simulink model "intento_50metrosporsegundo"  (R2024b)
settings: Solver=VariableStepAuto  StartTime=0.0  StopTime=600  RelTol=1e-3
libraries: slpidlib x1
settings Model: Creator=aulasingenieria  LastModifiedBy=Lenovo 618918
settings DebuggingCC: AlgebraicLoopMsg=none
settings RTWCC: GPUComputeCapability=3.5

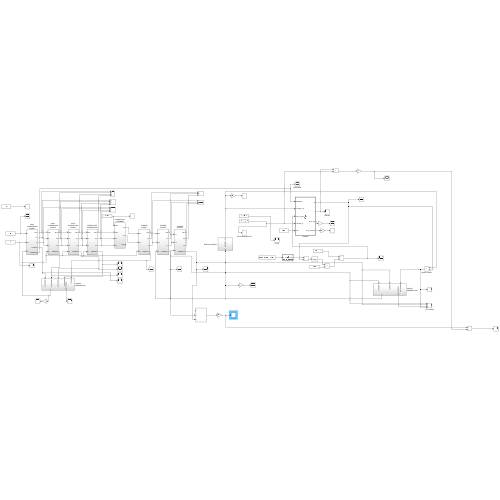
[thumbnail: Simulink's stored preview of the top-level diagram]
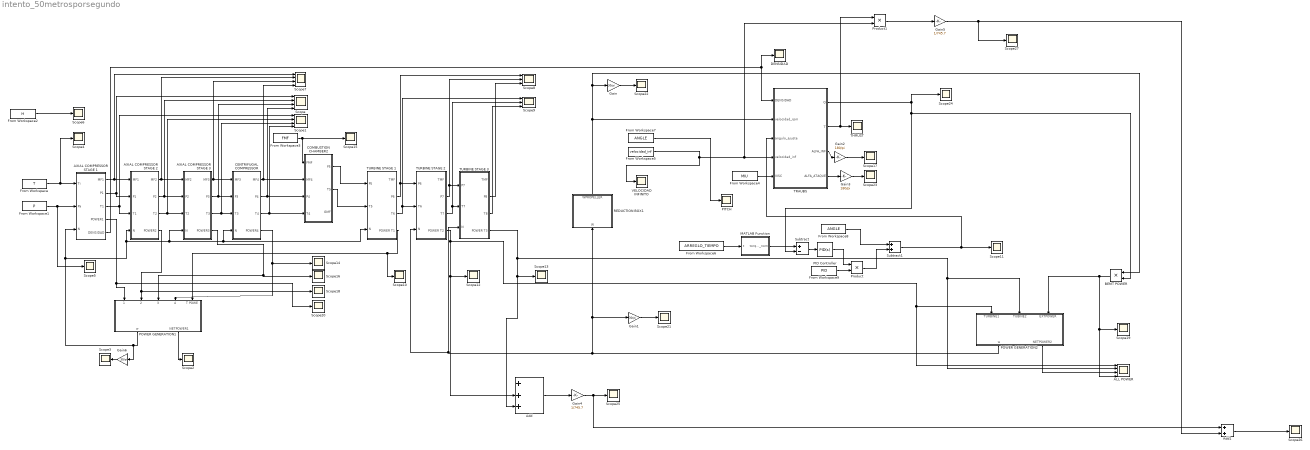
== system intento_50metrosporsegundo ==
  ALL POWER : Scope  NumInputPorts=4
  AXIAL COMPRESSOR STAGE 1 : Subsystem
  AXIAL COMPRESSOR STAGE 2 : Subsystem
  AXIAL COMPRESSOR STAGE 3 : Subsystem
  Add : Sum  Inputs=+++
  Add1 : Sum
  BEMT POWER : Product
  CENTRIFUGAL COMPRESSOR : Subsystem
  COMBUSTION CHAMBER2 : Subsystem
  DENSIDAD : Scope
  From Workspace : FromWorkspace  VariableName=T
  From Workspace1 : FromWorkspace  VariableName=P
  From Workspace2 : FromWorkspace  VariableName=H
  From Workspace3 : FromWorkspace  VariableName=FMF
  From Workspace4 : FromWorkspace  VariableName=MIU
  From Workspace5 : FromWorkspace  VariableName=velocidad_inf
  From Workspace6 : FromWorkspace  VariableName=ARREGLO_TIEMPO
  From Workspace7 : FromWorkspace  VariableName=ANGLE
  From Workspace8 : FromWorkspace  VariableName=ANGLE
  From Workspace9 : FromWorkspace  VariableName=PID
  Gain : Gain  Gain=30/pi
  Gain1 : Gain  Gain=30/pi
  Gain2 : Gain  Gain=180/pi
  Gain3 : Gain  Gain=180/pi
  Gain4 : Gain  Gain=1/745.7
  Gain5 : Gain  Gain=1/745.7
  Gain6 : Gain  Gain=30/pi
  MATLAB Function : MATLAB Function  TreatAsAtomicUnit=on
  PID Controller : slpidlib/PID Controller  Controller=PID  Form=Parallel  TimeDomain=Continuous-time  UseExternalTs=off  SampleTime=-1  IntegratorMethod=Forward Euler  FilterMethod=Forward Euler  ControllerParametersSource=internal  P=0.001  I=0.0001  UseKiTs=off  D=0.0001  UseExternalDerivativeSource=off  N=100  UseFilter=on  TunerSelectOption=Transfer Function Based (PID Tuner App)  InitialConditionSource=internal  InitialConditionForIntegrator=0  InitialConditionForFilter=0  DifferentiatorICPrevScaledInput=0  ExternalReset=none  TrackingMode=off  Kt=1  LimitOutput=off  SatLimitsSource=internal  UpperSaturationLimit=inf  LowerSaturationLimit=-inf  LinearizeAsGain=on  AntiWindupMode=none  Kb=1  LimitIntegrator=off  UpperIntegratorSaturationLimit=inf  LowerIntegratorSaturationLimit=-inf  POutMin=[]  POutMax=[]  IOutMin=[]  IOutMax=[]  DOutMin=[]  DOutMax=[]  NOutMin=[]  NOutMax=[]  SumOutMin=[]  SumOutMax=[]  SaturationOutMin=[]  SaturationOutMax=[]  PParamMin=[]  PParamMax=[]  IParamMin=[]  IParamMax=[]  DParamMin=[]  DParamMax=[]  NParamMin=[]  NParamMax=[]  KbParamMin=[]  KbParamMax=[]  KtParamMin=[]  KtParamMax=[]  KbOutMin=[]  KbOutMax=[]  KtOutMin=[]  KtOutMax=[]  IntegratorOutMin=[]  IntegratorOutMax=[]  FilterOutMin=[]  FilterOutMax=[]  SumI1OutMin=[]  SumI1OutMax=[]  SumI2OutMin=[]  SumI2OutMax=[]  SumI3OutMin=[]  SumI3OutMax=[]  SumI4OutMin=[]  SumI4OutMax=[]  SumDOutMin=[]  SumDOutMax=[]  DifferentiatorOutMin=[]  DifferentiatorOutMax=[]  FilterDiffOutCoefMin=[]  FilterDiffOutCoefMax=[]  ReciprocalOutMin=[]  ReciprocalOutMax=[]  SumDenOutMin=[]  SumDenOutMax=[]  SumNumOutMin=[]  SumNumOutMax=[]  DivideOutMin=[]  DivideOutMax=[]  UdiffTsProdOutMin=[]  UdiffTsProdOutMax=[]  NTsProdOutMin=[]  NTsProdOutMax=[]  UintegralTsProdOutMin=[]  UintegralTsProdOutMax=[]  UngainTsProdOutMin=[]  UngainTsProdOutMax=[]  ClampingZeroOutDataTypeStr=Inherit: Inherit via back propagation  ClampingZeroOutMin=[]  ClampingZeroOutMax=[]  FilterDenConstantOutDataTypeStr=Inherit: Inherit via back propagation  FilterDenConstantOutMin=[]  FilterDenConstantOutMax=[]  PCopyOutDataTypeStr=Inherit: Inherit via back propagation  PCopyOutMin=[]  PCopyOutMax=[]  NCopyOutDataTypeStr=Inherit: Inherit via back propagation  NCopyOutMin=[]  NCopyOutMax=[]  IntegratorContinuousStateAttributes=''  IntegratorStateMustResolveToSignalObject=off  IntegratorRTWStateStorageClass=Auto  FilterContinuousStateAttributes=''  FilterStateMustResolveToSignalObject=off  FilterRTWStateStorageClass=Auto  ParallelPVariant=InternalParameters  IdealPVariant=Disabled  IVariant=InternalParameters  DVariant=InternalParameters  IntegratorVariant=Continuous  SatVariant=Disabled  AWVariant=Passthrough  PCopyVariant=Disabled  TRVariant=Disabled  FdbkBlocksVariant=Forward  IdealPFdbkVariant=Disabled  SatFdbkVariant=Disabled  DerivativeFilterVariant=ContFilter  NVariant=InternalParameters  NCopyVariant=Disabled  FilterICVariant=InternalICsFilter  IntegratorICVariant=InternalICs  ExternalResetVariant=Disabled  TRSumVariant=Passthrough  SumFdbkVariant=Disabled  SumVariant=Sum_PID  TsampFilterVariant=InternalTs  TsampNgainVariant=Passthrough  TsampIntegralVariant=Disabled_SignalSpec  ExternalSaturationOutDataTypeStr=Inherit: Same as second input  DerivativeSourceVariant=ErrorSignal  PreIntVariant=InternalPreInt
  PITCH : Scope
  POWER GENERATION1 : Subsystem
  POWER GENERATION2 : Subsystem
  Product : Product
  Product1 : Product
  REDUCTION BOX1 : Subsystem
  Scope : Scope  NumInputPorts=4
  Scope1 : Scope  NumInputPorts=4
  Scope{2..6,10..27} (23 alike) : Scope
  Scope7 : Scope  NumInputPorts=4
  Scope8 : Scope  NumInputPorts=3
  Scope9 : Scope  NumInputPorts=3
  Subtract : Sum  Inputs=+-
  Subtract1 : Sum
  THRUST : Scope
  TRAUBS : MATLAB Function  TreatAsAtomicUnit=on
  TURBINE STAGE 1 : Subsystem
  TURBINE STAGE 2 : Subsystem
  TURBINE STAGE 3 : Subsystem
  VELOCIDAD INFINITO : Scope
  wires:
  TURBINE STAGE 1/2(P6) -> Scope8/1, TURBINE STAGE 2/1(P6)
  TURBINE STAGE 2/3(T7) -> TURBINE STAGE 3/2(T7), Scope9/2
  AXIAL COMPRESSOR STAGE 3/3(T3) -> CENTRIFUGAL COMPRESSOR/3(T3), Scope1/3
  CENTRIFUGAL COMPRESSOR/4(POWER4) -> POWER GENERATION1/4(CC POWER), Scope14/1
  CENTRIFUGAL COMPRESSOR/2(P4) -> COMBUSTION CHAMBER2/3(P4), Scope/4
  TURBINE STAGE 2/2(P7) -> Scope8/2, TURBINE STAGE 3/1(P7)
  TURBINE STAGE 3/2(P8) -> Scope8/3
  AXIAL COMPRESSOR STAGE 3/1(MF3) -> CENTRIFUGAL COMPRESSOR/1(MF3), Scope7/3
  TURBINE STAGE 3/3(T8) -> Scope9/3
  CENTRIFUGAL COMPRESSOR/3(T4) -> COMBUSTION CHAMBER2/4(T4), Scope1/4
  AXIAL COMPRESSOR STAGE 2/2(P2) -> AXIAL COMPRESSOR STAGE 3/2(P2), Scope/2
  TURBINE STAGE 1/3(T6) -> TURBINE STAGE 2/2(T6), Scope9/1
  POWER GENERATION1/1(w) -> Gain6/1, AXIAL COMPRESSOR STAGE 1/3(N), AXIAL COMPRESSOR STAGE 3/4(N), CENTRIFUGAL COMPRESSOR/4(N), TURBINE STAGE 1/3(N), AXIAL COMPRESSOR STAGE 2/4(N)
  AXIAL COMPRESSOR STAGE 3/2(P3) -> CENTRIFUGAL COMPRESSOR/2(P3), Scope/3
  From Workspace1/1 -> Scope5/1, AXIAL COMPRESSOR STAGE 1/2(Pa)
  CENTRIFUGAL COMPRESSOR/1(MF4) -> Scope7/4, COMBUSTION CHAMBER2/2(MF4)
  COMBUSTION CHAMBER2/1(P5) -> TURBINE STAGE 1/1(P5)
  POWER GENERATION1/2(NETPOWER1) -> Scope2/1
  AXIAL COMPRESSOR STAGE 2/1(MF2) -> AXIAL COMPRESSOR STAGE 3/1(MF2), Scope7/2
  From Workspace3/1 -> Scope15/1, COMBUSTION CHAMBER2/1(FMF)
  AXIAL COMPRESSOR STAGE 3/4(POWER3) -> Scope16/1, POWER GENERATION1/3(AC POWER3)
  AXIAL COMPRESSOR STAGE 2/3(T2) -> AXIAL COMPRESSOR STAGE 3/3(T2), Scope1/2
  TURBINE STAGE 1/4(POWER T1) -> Scope10/1, POWER GENERATION1/5(T POWE)
  AXIAL COMPRESSOR STAGE 1/2(P1) -> AXIAL COMPRESSOR STAGE 2/2(P1), Scope/1
  AXIAL COMPRESSOR STAGE 1/1(MF1) -> AXIAL COMPRESSOR STAGE 2/1(MF1), Scope7/1
  AXIAL COMPRESSOR STAGE 2/4(POWER2) -> Scope18/1, POWER GENERATION1/2(AC POWER2)
  From Workspace/1 -> Scope4/1, AXIAL COMPRESSOR STAGE 1/1(Ti)
  AXIAL COMPRESSOR STAGE 1/4(POWER1) -> Scope20/1, POWER GENERATION1/1(AC POWER1)
  AXIAL COMPRESSOR STAGE 1/3(T1) -> AXIAL COMPRESSOR STAGE 2/3(T1), Scope1/1
  COMBUSTION CHAMBER2/2(T5) -> TURBINE STAGE 1/2(T5)
  From Workspace2/1 -> Scope6/1
  TURBINE STAGE 2/4(POWER T2) -> Scope12/1, Add/2, ALL POWER/1, POWER GENERATION2/1(TURBINE1)
  TURBINE STAGE 3/4(POWER T3) -> Add/3, Scope13/1, ALL POWER/2, POWER GENERATION2/2(TUBINE2)
  From Workspace5/1 -> Product1/2, TRAUBS/4(velocidad_inf), VELOCIDAD INFINITO/1
  POWER GENERATION2/2(NETPOWER2) -> ALL POWER/3
  Gain/1 -> Scope22/1
  REDUCTION BOX1/1(WPROPELLER) -> BEMT POWER/1, Gain/1, TRAUBS/2(velocidad_rpm)
  BEMT POWER/1 -> POWER GENERATION2/3(EXTPOWER), Scope19/1, ALL POWER/4
  AXIAL COMPRESSOR STAGE 1/5(DENSIDAD) -> DENSIDAD/1, TRAUBS/1(DENSIDAD)
  From Workspace4/1 -> TRAUBS/5(VISC)
  Subtract/1 -> PID Controller/1
  MATLAB Function/1(torque_nom) -> Subtract/1
  From Workspace6/1 -> MATLAB Function/1(t)
  From Workspace8/1 -> Subtract1/1
  POWER GENERATION2/1(w) -> Gain1/1, REDUCTION BOX1/1(W), TURBINE STAGE 3/3(N), TURBINE STAGE 2/3(N)
  From Workspace7/1 -> PITCH/1
  TRAUBS/1(Q) -> Scope24/1, BEMT POWER/2, Subtract/2
  TRAUBS/2(T) -> Product1/1, THRUST/1
  From Workspace9/1 -> Product/2
  PID Controller/1 -> Product/1
  Product/1 -> Subtract1/2
  Gain1/1 -> Scope21/1
  TRAUBS/3(ALFA_INF) -> Gain2/1
  Gain2/1 -> Scope17/1
  TRAUBS/4(ALFA_ATAQUE) -> Gain3/1
  Gain3/1 -> Scope23/1
  Subtract1/1 -> TRAUBS/3(angulo_ajuste), Scope11/1
  Gain4/1 -> Scope25/1, Add1/1
  Add/1 -> Gain4/1
  Product1/1 -> Gain5/1
  Gain5/1 -> Scope27/1, Add1/2
  Add1/1 -> Scope26/1
  Gain6/1 -> Scope3/1

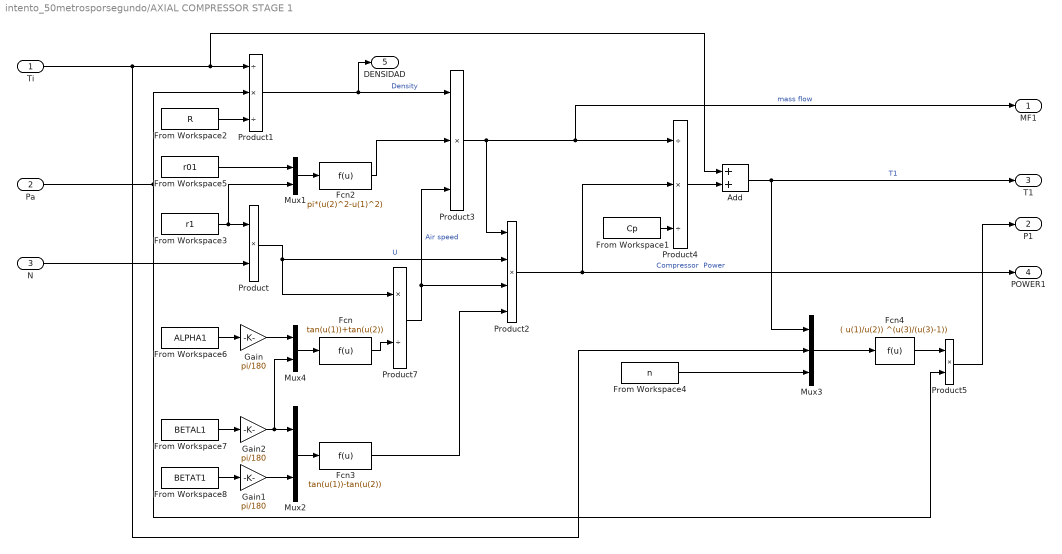
== system intento_50metrosporsegundo/AXIAL COMPRESSOR STAGE 1 ==
  Ti : Inport
  Pa : Inport  Port=2
  N : Inport  Port=3
  Add : Sum
  Fcn : Fcn  Expr=tan(u(1))+tan(u(2))
  Fcn2 : Fcn  Expr=pi*(u(2)^2-u(1)^2)
  Fcn3 : Fcn  Expr=tan(u(1))-tan(u(2))
  Fcn4 : Fcn  Expr=( u(1)/u(2)) ^(u(3)/(u(3)-1))
  From Workspace1 : FromWorkspace  VariableName=Cp
  From Workspace2 : FromWorkspace  VariableName=R
  From Workspace3 : FromWorkspace  VariableName=r1
  From Workspace4 : FromWorkspace  VariableName=n
  From Workspace5 : FromWorkspace  VariableName=r01
  From Workspace6 : FromWorkspace  VariableName=ALPHA1
  From Workspace7 : FromWorkspace  VariableName=BETAL1
  From Workspace8 : FromWorkspace  VariableName=BETAT1
  Gain : Gain  Gain=pi/180
  Gain1 : Gain  Gain=pi/180
  Gain2 : Gain  Gain=pi/180
  Mux1 : Mux  Inputs=2
  Mux2 : Mux  Inputs=2
  Mux3 : Mux  Inputs=3
  Mux4 : Mux  Inputs=2
  Product : Product
  Product1 : Product  Inputs=/*/
  Product2 : Product  Inputs=****
  Product3 : Product  Inputs=3
  Product4 : Product  Inputs=/*/
  Product5 : Product
  Product7 : Product  Inputs=*/
  MF1 : Outport
  P1 : Outport  Port=2
  T1 : Outport  Port=3
  POWER1 : Outport  Port=4
  DENSIDAD : Outport  Port=5
  wires:
  Fcn3/1 -> Product2/4
  From Workspace1/1 -> Product4/3
  Ti/1 -> Add/1, Product1/1, Mux3/2
  Mux3/1 -> Fcn4/1
  From Workspace8/1 -> Gain1/1
  Product1/1 -> DENSIDAD/1, Product3/1  "Density"
  Gain/1 -> Mux4/1
  From Workspace4/1 -> Mux3/3
  Mux1/1 -> Fcn2/1
  Mux2/1 -> Fcn3/1
  Product7/1 -> Product2/3, Product3/3  "Air speed"
  Product/1 -> Product7/1, Product2/2  "U"
  Product3/1 -> Product4/1, MF1/1, Product2/1  "mass flow"
  Fcn2/1 -> Product3/2
  Gain1/1 -> Mux2/2
  From Workspace6/1 -> Gain/1
  From Workspace5/1 -> Mux1/1
  N/1 -> Product/2
  From Workspace7/1 -> Gain2/1
  From Workspace3/1 -> Mux1/2, Product/1
  Add/1 -> T1/1, Mux3/1  "T1"
  Product4/1 -> Add/2
  From Workspace2/1 -> Product1/3
  Gain2/1 -> Mux2/1, Mux4/2
  Product2/1 -> POWER1/1, Product4/2  "Compressor  Power"
  Mux4/1 -> Fcn/1
  Product5/1 -> P1/1
  Fcn4/1 -> Product5/1
  Fcn/1 -> Product7/2
  Pa/1 -> Product1/2, Product5/2

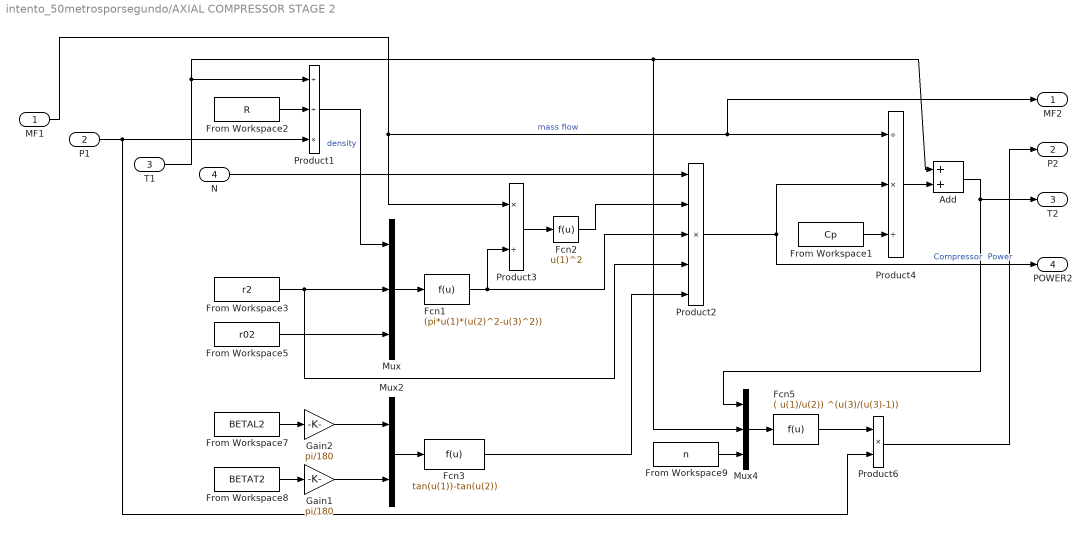
== system intento_50metrosporsegundo/AXIAL COMPRESSOR STAGE 2 ==
  MF1 : Inport
  P1 : Inport  Port=2
  T1 : Inport  Port=3
  N : Inport  Port=4
  Add : Sum
  Fcn1 : Fcn  Expr=(pi*u(1)*(u(2)^2-u(3)^2))
  Fcn2 : Fcn  Expr=u(1)^2
  Fcn3 : Fcn  Expr=tan(u(1))-tan(u(2))
  Fcn5 : Fcn  Expr=( u(1)/u(2)) ^(u(3)/(u(3)-1))
  From Workspace1 : FromWorkspace  VariableName=Cp
  From Workspace2 : FromWorkspace  VariableName=R
  From Workspace3 : FromWorkspace  VariableName=r2
  From Workspace5 : FromWorkspace  VariableName=r02
  From Workspace7 : FromWorkspace  VariableName=BETAL2
  From Workspace8 : FromWorkspace  VariableName=BETAT2
  From Workspace9 : FromWorkspace  VariableName=n
  Gain1 : Gain  Gain=pi/180
  Gain2 : Gain  Gain=pi/180
  Mux : Mux  Inputs=3
  Mux2 : Mux  Inputs=2
  Mux4 : Mux  Inputs=3
  Product1 : Product  Inputs=//*
  Product2 : Product  Inputs=*****
  Product3 : Product  Inputs=*/
  Product4 : Product  Inputs=/*/
  Product6 : Product
  MF2 : Outport
  P2 : Outport  Port=2
  T2 : Outport  Port=3
  POWER2 : Outport  Port=4
  wires:
  Add/1 -> T2/1, Mux4/1
  Product4/1 -> Add/2
  From Workspace3/1 -> Product2/4, Mux/2
  P1/1 -> Product1/3, Product6/2
  Product2/1 -> POWER2/1, Product4/2  "Compressor  Power"
  MF1/1 -> Product3/1, MF2/1, Product4/1  "mass flow"
  From Workspace5/1 -> Mux/3
  T1/1 -> Product1/1, Mux4/2, Add/1
  Fcn3/1 -> Product2/5
  From Workspace7/1 -> Gain2/1
  From Workspace1/1 -> Product4/3
  Gain2/1 -> Mux2/1
  Mux2/1 -> Fcn3/1
  Gain1/1 -> Mux2/2
  From Workspace8/1 -> Gain1/1
  From Workspace2/1 -> Product1/2
  Product1/1 -> Mux/1  "density"
  Fcn2/1 -> Product2/2
  Mux/1 -> Fcn1/1
  Fcn1/1 -> Product2/3, Product3/2
  Product3/1 -> Fcn2/1
  N/1 -> Product2/1
  Fcn5/1 -> Product6/1
  Mux4/1 -> Fcn5/1
  Product6/1 -> P2/1
  From Workspace9/1 -> Mux4/3

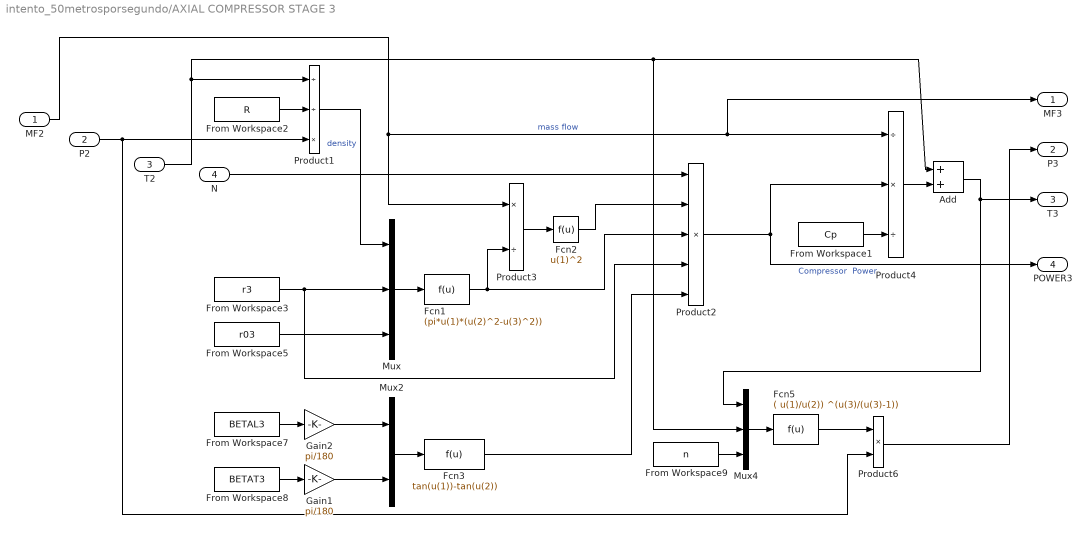
== system intento_50metrosporsegundo/AXIAL COMPRESSOR STAGE 3 ==
  MF2 : Inport
  P2 : Inport  Port=2
  T2 : Inport  Port=3
  N : Inport  Port=4
  Add : Sum
  Fcn1 : Fcn  Expr=(pi*u(1)*(u(2)^2-u(3)^2))
  Fcn2 : Fcn  Expr=u(1)^2
  Fcn3 : Fcn  Expr=tan(u(1))-tan(u(2))
  Fcn5 : Fcn  Expr=( u(1)/u(2)) ^(u(3)/(u(3)-1))
  From Workspace1 : FromWorkspace  VariableName=Cp
  From Workspace2 : FromWorkspace  VariableName=R
  From Workspace3 : FromWorkspace  VariableName=r3
  From Workspace5 : FromWorkspace  VariableName=r03
  From Workspace7 : FromWorkspace  VariableName=BETAL3
  From Workspace8 : FromWorkspace  VariableName=BETAT3
  From Workspace9 : FromWorkspace  VariableName=n
  Gain1 : Gain  Gain=pi/180
  Gain2 : Gain  Gain=pi/180
  Mux : Mux  Inputs=3
  Mux2 : Mux  Inputs=2
  Mux4 : Mux  Inputs=3
  Product1 : Product  Inputs=//*
  Product2 : Product  Inputs=*****
  Product3 : Product  Inputs=*/
  Product4 : Product  Inputs=/*/
  Product6 : Product
  MF3 : Outport
  P3 : Outport  Port=2
  T3 : Outport  Port=3
  POWER3 : Outport  Port=4
  wires:
  Add/1 -> T3/1, Mux4/1
  Product4/1 -> Add/2
  From Workspace3/1 -> Product2/4, Mux/2
  P2/1 -> Product1/3, Product6/2
  Product2/1 -> POWER3/1, Product4/2  "Compressor  Power"
  MF2/1 -> Product3/1, MF3/1, Product4/1  "mass flow"
  From Workspace5/1 -> Mux/3
  T2/1 -> Product1/1, Mux4/2, Add/1
  Fcn3/1 -> Product2/5
  From Workspace7/1 -> Gain2/1
  From Workspace1/1 -> Product4/3
  Gain2/1 -> Mux2/1
  Mux2/1 -> Fcn3/1
  Gain1/1 -> Mux2/2
  From Workspace8/1 -> Gain1/1
  From Workspace2/1 -> Product1/2
  Product1/1 -> Mux/1  "density"
  Fcn2/1 -> Product2/2
  Mux/1 -> Fcn1/1
  Fcn1/1 -> Product2/3, Product3/2
  Product3/1 -> Fcn2/1
  N/1 -> Product2/1
  Fcn5/1 -> Product6/1
  Mux4/1 -> Fcn5/1
  Product6/1 -> P3/1
  From Workspace9/1 -> Mux4/3

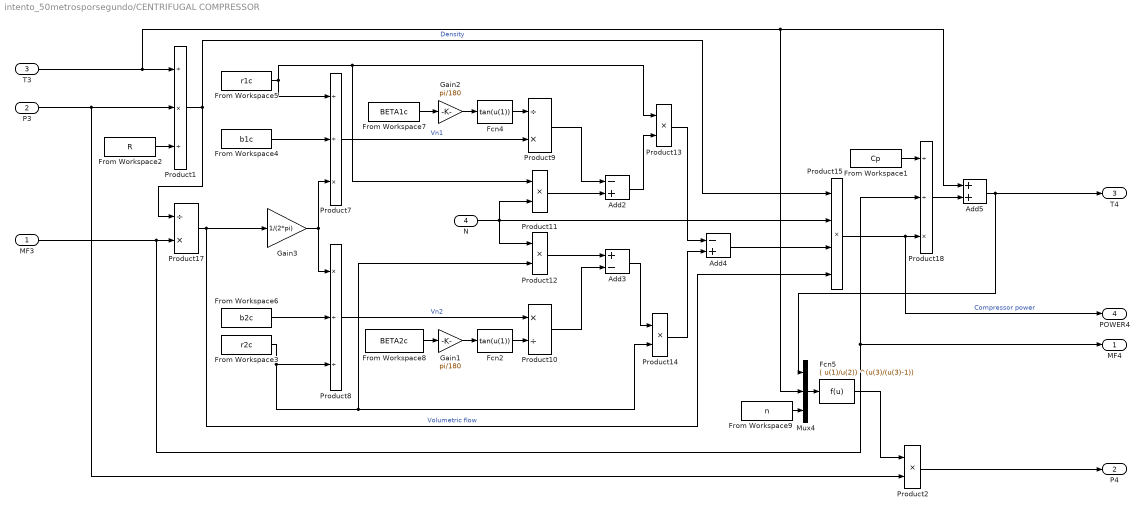
== system intento_50metrosporsegundo/CENTRIFUGAL COMPRESSOR ==
  MF3 : Inport
  P3 : Inport  Port=2
  T3 : Inport  Port=3
  N : Inport  Port=4
  Add2 : Sum  Inputs=-+
  Add3 : Sum  Inputs=+-
  Add4 : Sum  Inputs=-+
  Add5 : Sum  Inputs=2
  Fcn2 : Fcn  Expr=tan(u(1))
  Fcn4 : Fcn  Expr=tan(u(1))
  Fcn5 : Fcn  Expr=( u(1)/u(2)) ^(u(3)/(u(3)-1))
  From Workspace1 : FromWorkspace  VariableName=Cp
  From Workspace2 : FromWorkspace  VariableName=R
  From Workspace3 : FromWorkspace  VariableName=r2c
  From Workspace4 : FromWorkspace  VariableName=b1c
  From Workspace5 : FromWorkspace  VariableName=r1c
  From Workspace6 : FromWorkspace  VariableName=b2c
  From Workspace7 : FromWorkspace  VariableName=BETA1c
  From Workspace8 : FromWorkspace  VariableName=BETA2c
  From Workspace9 : FromWorkspace  VariableName=n
  Gain1 : Gain  Gain=pi/180
  Gain2 : Gain  Gain=pi/180
  Gain3 : Gain  Gain=1/(2*pi)
  Mux4 : Mux  Inputs=3
  Product1 : Product  Inputs=/*/
  Product10 : Product  Inputs=*/
  Product{2,11..14} (5 alike) : Product
  Product15 : Product  Inputs=4
  Product17 : Product  Inputs=/*
  Product18 : Product  Inputs=//*
  Product7 : Product  Inputs=//*
  Product8 : Product  Inputs=*//
  Product9 : Product  Inputs=/*
  MF4 : Outport
  P4 : Outport  Port=2
  T4 : Outport  Port=3
  POWER4 : Outport  Port=4
  wires:
  From Workspace2/1 -> Product1/3
  P3/1 -> Product1/2, Product2/2
  T3/1 -> Product1/1, Mux4/2, Add5/1
  From Workspace8/1 -> Gain1/1
  From Workspace7/1 -> Gain2/1
  From Workspace4/1 -> Product7/2
  From Workspace5/1 -> Product13/1, Product11/1, Product7/1
  Product1/1 -> Product15/1, Product17/1  "Density"
  From Workspace6/1 -> Product8/2
  Gain1/1 -> Fcn2/1
  Gain2/1 -> Fcn4/1
  Fcn4/1 -> Product9/1
  Product7/1 -> Product9/2  "Vn1"
  Product8/1 -> Product10/1  "Vn2"
  Fcn2/1 -> Product10/2
  Product10/1 -> Add3/2
  Product9/1 -> Add2/1
  N/1 -> Product12/1, Product15/2, Product11/2
  Product11/1 -> Add2/2
  Product12/1 -> Add3/1
  Add2/1 -> Product13/2
  Add3/1 -> Product14/1
  From Workspace3/1 -> Product12/2, Product14/2, Product8/3
  Product13/1 -> Add4/1
  Product14/1 -> Add4/2
  Add4/1 -> Product15/3
  Product17/1 -> Product15/4, Gain3/1  "Volumetric flow"
  MF3/1 -> Product18/2, MF4/1, Product17/2
  Gain3/1 -> Product7/3, Product8/1
  Product2/1 -> P4/1
  Product15/1 -> POWER4/1, Product18/3  "Compressor power"
  Product18/1 -> Add5/2
  From Workspace1/1 -> Product18/1
  Add5/1 -> Mux4/1, T4/1
  Mux4/1 -> Fcn5/1
  From Workspace9/1 -> Mux4/3
  Fcn5/1 -> Product2/1

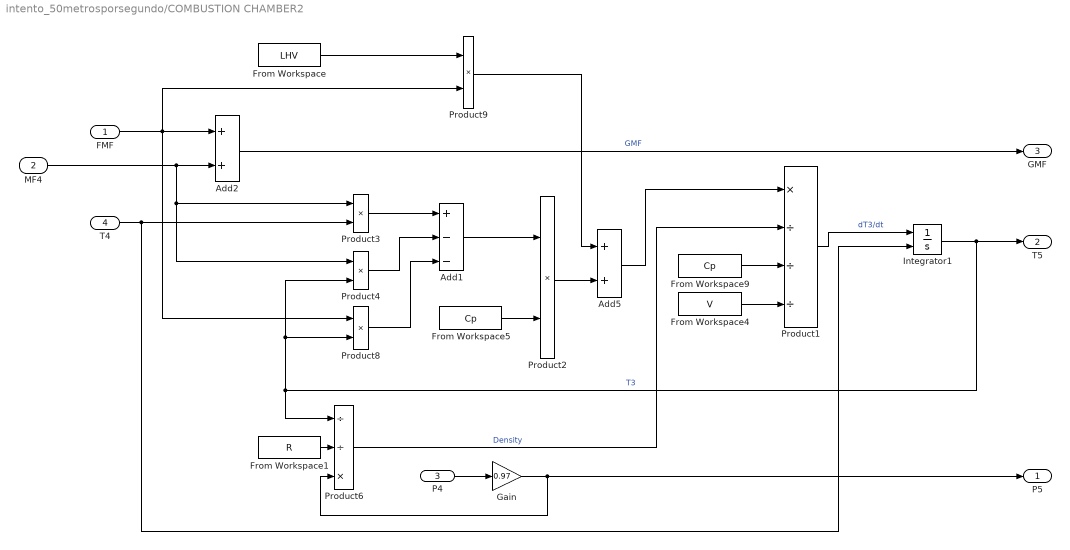
== system intento_50metrosporsegundo/COMBUSTION CHAMBER2 ==
  FMF : Inport
  MF4 : Inport  Port=2
  P4 : Inport  Port=3
  T4 : Inport  Port=4
  Add1 : Sum  Inputs=+--
  Add2 : Sum  Inputs=2
  Add5 : Sum  Inputs=2
  From Workspace : FromWorkspace  VariableName=LHV
  From Workspace1 : FromWorkspace  VariableName=R
  From Workspace4 : FromWorkspace  VariableName=V
  From Workspace5 : FromWorkspace  VariableName=Cp
  From Workspace9 : FromWorkspace  VariableName=Cp
  Gain : Gain  Gain=0.97
  Integrator1 : Integrator  InitialConditionSource=external
  Product1 : Product  Inputs=*///
  Product{2..4,8..9} (5 alike) : Product
  Product6 : Product  Inputs=//*
  P5 : Outport
  T5 : Outport  Port=2
  GMF : Outport  Port=3
  wires:
  T4/1 -> Integrator1/2, Product3/2
  Product6/1 -> Product1/2  "Density"
  MF4/1 -> Add2/2, Product3/1, Product4/1
  FMF/1 -> Add2/1, Product9/2, Product8/1
  From Workspace/1 -> Product9/1
  From Workspace4/1 -> Product1/4
  From Workspace9/1 -> Product1/3
  From Workspace5/1 -> Product2/2
  Add1/1 -> Product2/1
  Product3/1 -> Add1/1
  Product4/1 -> Add1/2
  Integrator1/1 -> Product6/1, Product8/2, Product4/2, T5/1  "T3"
  Product8/1 -> Add1/3
  Product9/1 -> Add5/1
  Product2/1 -> Add5/2
  Add5/1 -> Product1/1
  Product1/1 -> Integrator1/1  "dT3/dt"
  From Workspace1/1 -> Product6/2
  Gain/1 -> Product6/3, P5/1
  P4/1 -> Gain/1
  Add2/1 -> GMF/1  "GMF"

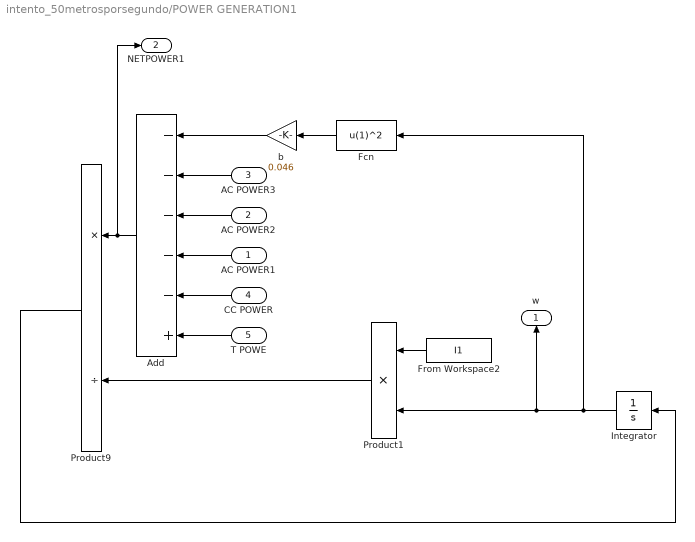
== system intento_50metrosporsegundo/POWER GENERATION1 ==
  AC POWER1 : Inport
  AC POWER2 : Inport  Port=2
  AC POWER3 : Inport  Port=3
  CC POWER : Inport  Port=4
  T POWE : Inport  Port=5
  Add : Sum  Inputs=-----+
  Fcn : Fcn  Expr=u(1)^2
  From Workspace2 : FromWorkspace  VariableName=I1
  Integrator : Integrator  InitialCondition=1256
  Product1 : Product
  Product9 : Product  Inputs=*/
  b : Gain  Gain=0.046
  w : Outport
  NETPOWER1 : Outport  Port=2
  wires:
  Product1/1 -> Product9/2
  Add/1 -> NETPOWER1/1, Product9/1
  Product9/1 -> Integrator/1
  T POWE/1 -> Add/6
  AC POWER1/1 -> Add/4
  AC POWER2/1 -> Add/3
  AC POWER3/1 -> Add/2
  CC POWER/1 -> Add/5
  From Workspace2/1 -> Product1/1
  Integrator/1 -> Fcn/1, Product1/2, w/1
  Fcn/1 -> b/1
  b/1 -> Add/1

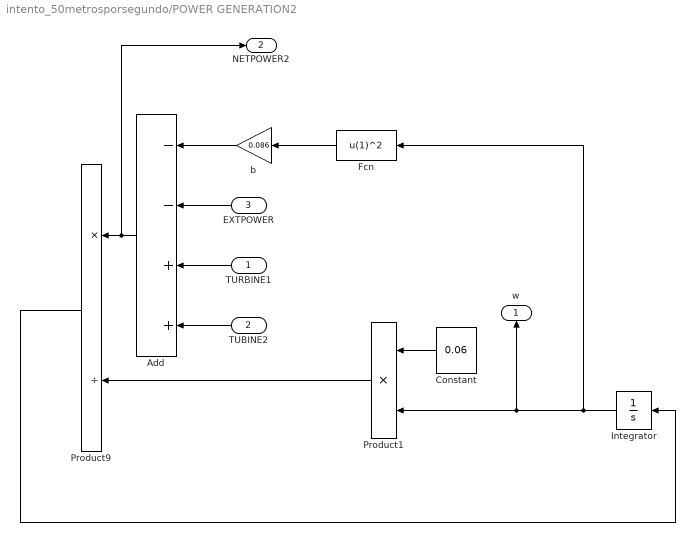
== system intento_50metrosporsegundo/POWER GENERATION2 ==
  TURBINE1 : Inport
  TUBINE2 : Inport  Port=2
  EXTPOWER : Inport  Port=3
  Add : Sum  Inputs=--++
  Constant : Constant  Value=0.06
  Fcn : Fcn  Expr=u(1)^2
  Integrator : Integrator  InitialCondition=90
  Product1 : Product
  Product9 : Product  Inputs=*/
  b : Gain  Gain=0.086
  w : Outport  VectorParamsAs1DForOutWhenUnconnected=off
  NETPOWER2 : Outport  Port=2  VectorParamsAs1DForOutWhenUnconnected=off
  wires:
  Product1/1 -> Product9/2
  Add/1 -> NETPOWER2/1, Product9/1
  Product9/1 -> Integrator/1
  TUBINE2/1 -> Add/4
  TURBINE1/1 -> Add/3
  Constant/1 -> Product1/1
  Integrator/1 -> Fcn/1, Product1/2, w/1
  Fcn/1 -> b/1
  b/1 -> Add/1
  EXTPOWER/1 -> Add/2

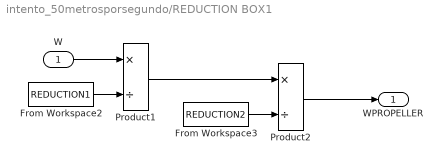
== system intento_50metrosporsegundo/REDUCTION BOX1 ==
  W : Inport
  From Workspace2 : FromWorkspace  VariableName=REDUCTION1
  From Workspace3 : FromWorkspace  VariableName=REDUCTION2
  Product1 : Product  Inputs=*/
  Product2 : Product  Inputs=*/
  WPROPELLER : Outport
  wires:
  W/1 -> Product1/1
  Product2/1 -> WPROPELLER/1
  Product1/1 -> Product2/1
  From Workspace3/1 -> Product2/2
  From Workspace2/1 -> Product1/2

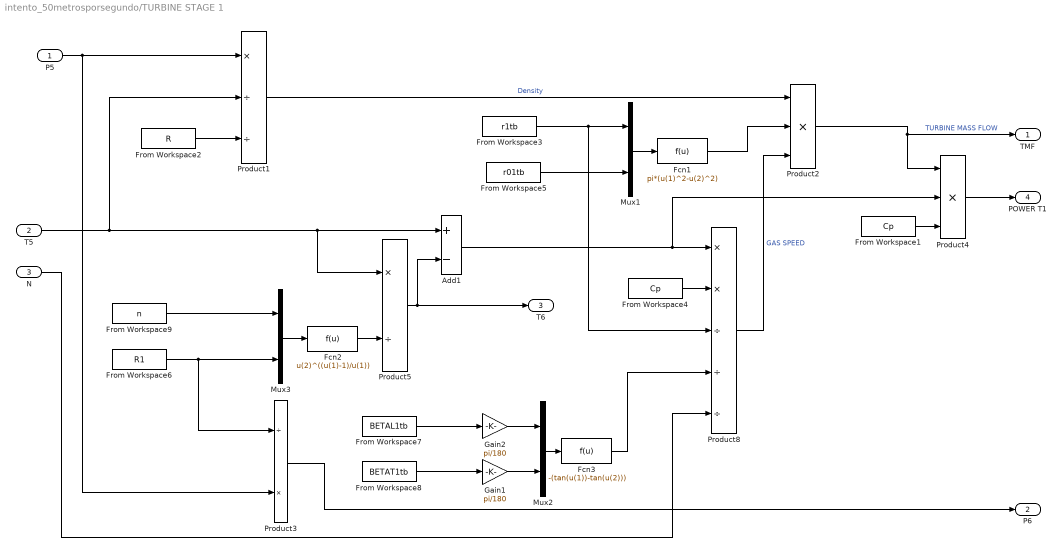
== system intento_50metrosporsegundo/TURBINE STAGE 1 ==
  P5 : Inport
  T5 : Inport  Port=2
  N : Inport  Port=3
  Add1 : Sum  Inputs=+-
  Fcn1 : Fcn  Expr=pi*(u(1)^2-u(2)^2)
  Fcn2 : Fcn  Expr=u(2)^((u(1)-1)/u(1))
  Fcn3 : Fcn  Expr=-(tan(u(1))-tan(u(2)))
  From Workspace1 : FromWorkspace  VariableName=Cp
  From Workspace2 : FromWorkspace  VariableName=R
  From Workspace3 : FromWorkspace  VariableName=r1tb
  From Workspace4 : FromWorkspace  VariableName=Cp
  From Workspace5 : FromWorkspace  VariableName=r01tb
  From Workspace6 : FromWorkspace  VariableName=R1
  From Workspace7 : FromWorkspace  VariableName=BETAL1tb
  From Workspace8 : FromWorkspace  VariableName=BETAT1tb
  From Workspace9 : FromWorkspace  VariableName=n
  Gain1 : Gain  Gain=pi/180
  Gain2 : Gain  Gain=pi/180
  Mux1 : Mux  Inputs=2
  Mux2 : Mux  Inputs=2
  Mux3 : Mux  Inputs=2
  Product1 : Product  Inputs=*//
  Product2 : Product  Inputs=3
  Product3 : Product  Inputs=/*
  Product4 : Product  Inputs=3
  Product5 : Product  Inputs=*/
  Product8 : Product  Inputs=**///
  TMF : Outport
  P6 : Outport  Port=2
  T6 : Outport  Port=3
  POWER T1 : Outport  Port=4
  wires:
  From Workspace3/1 -> Product8/3, Mux1/1
  Mux1/1 -> Fcn1/1
  Fcn1/1 -> Product2/2
  From Workspace5/1 -> Mux1/2
  Mux2/1 -> Fcn3/1
  Gain1/1 -> Mux2/2
  From Workspace8/1 -> Gain1/1
  From Workspace7/1 -> Gain2/1
  Gain2/1 -> Mux2/1
  From Workspace2/1 -> Product1/3
  P5/1 -> Product1/1, Product3/2
  Product3/1 -> P6/1
  From Workspace6/1 -> Product3/1, Mux3/2
  T5/1 -> Add1/1, Product5/1, Product1/2
  From Workspace9/1 -> Mux3/1
  Add1/1 -> Product4/2, Product8/1
  From Workspace4/1 -> Product8/2
  N/1 -> Product8/5
  Product8/1 -> Product2/3  "GAS SPEED"
  Product1/1 -> Product2/1  "Density"
  Product2/1 -> Product4/1, TMF/1  "TURBINE MASS FLOW"
  Mux3/1 -> Fcn2/1
  Fcn2/1 -> Product5/2
  From Workspace1/1 -> Product4/3
  Product4/1 -> POWER T1/1
  Product5/1 -> T6/1, Add1/2
  Fcn3/1 -> Product8/4

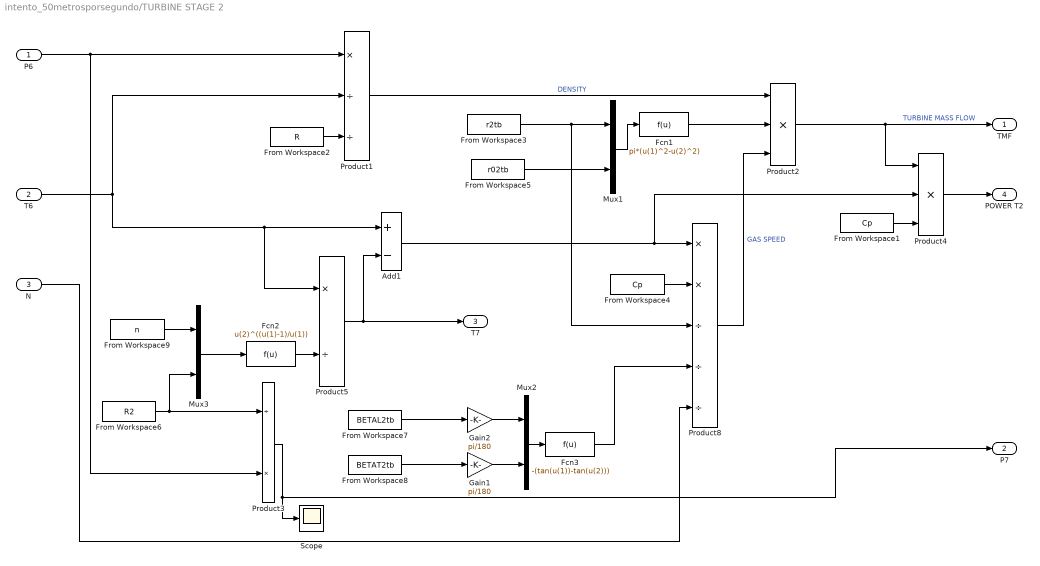
== system intento_50metrosporsegundo/TURBINE STAGE 2 ==
  P6 : Inport
  T6 : Inport  Port=2
  N : Inport  Port=3
  Add1 : Sum  Inputs=+-
  Fcn1 : Fcn  Expr=pi*(u(1)^2-u(2)^2)
  Fcn2 : Fcn  Expr=u(2)^((u(1)-1)/u(1))
  Fcn3 : Fcn  Expr=-(tan(u(1))-tan(u(2)))
  From Workspace1 : FromWorkspace  VariableName=Cp
  From Workspace2 : FromWorkspace  VariableName=R
  From Workspace3 : FromWorkspace  VariableName=r2tb
  From Workspace4 : FromWorkspace  VariableName=Cp
  From Workspace5 : FromWorkspace  VariableName=r02tb
  From Workspace6 : FromWorkspace  VariableName=R2
  From Workspace7 : FromWorkspace  VariableName=BETAL2tb
  From Workspace8 : FromWorkspace  VariableName=BETAT2tb
  From Workspace9 : FromWorkspace  VariableName=n
  Gain1 : Gain  Gain=pi/180
  Gain2 : Gain  Gain=pi/180
  Mux1 : Mux  Inputs=2
  Mux2 : Mux  Inputs=2
  Mux3 : Mux  Inputs=2
  Product1 : Product  Inputs=*//
  Product2 : Product  Inputs=3
  Product3 : Product  Inputs=/*
  Product4 : Product  Inputs=3
  Product5 : Product  Inputs=*/
  Product8 : Product  Inputs=**///
  Scope : Scope
  TMF : Outport
  P7 : Outport  Port=2
  T7 : Outport  Port=3
  POWER T2 : Outport  Port=4
  wires:
  From Workspace3/1 -> Mux1/1, Product8/3
  Mux1/1 -> Fcn1/1
  Fcn1/1 -> Product2/2
  From Workspace5/1 -> Mux1/2
  Mux2/1 -> Fcn3/1
  Gain1/1 -> Mux2/2
  From Workspace8/1 -> Gain1/1
  From Workspace7/1 -> Gain2/1
  Gain2/1 -> Mux2/1
  From Workspace2/1 -> Product1/3
  P6/1 -> Product1/1, Product3/2
  Product3/1 -> P7/1, Scope/1
  From Workspace6/1 -> Product3/1, Mux3/2
  T6/1 -> Product1/2, Add1/1, Product5/1
  From Workspace9/1 -> Mux3/1
  Product5/1 -> T7/1, Add1/2
  Add1/1 -> Product4/2, Product8/1
  From Workspace4/1 -> Product8/2
  N/1 -> Product8/5
  Product8/1 -> Product2/3  "GAS SPEED"
  Product1/1 -> Product2/1  "DENSITY"
  Product2/1 -> Product4/1, TMF/1  "TURBINE MASS FLOW"
  Mux3/1 -> Fcn2/1
  Fcn2/1 -> Product5/2
  From Workspace1/1 -> Product4/3
  Product4/1 -> POWER T2/1
  Fcn3/1 -> Product8/4

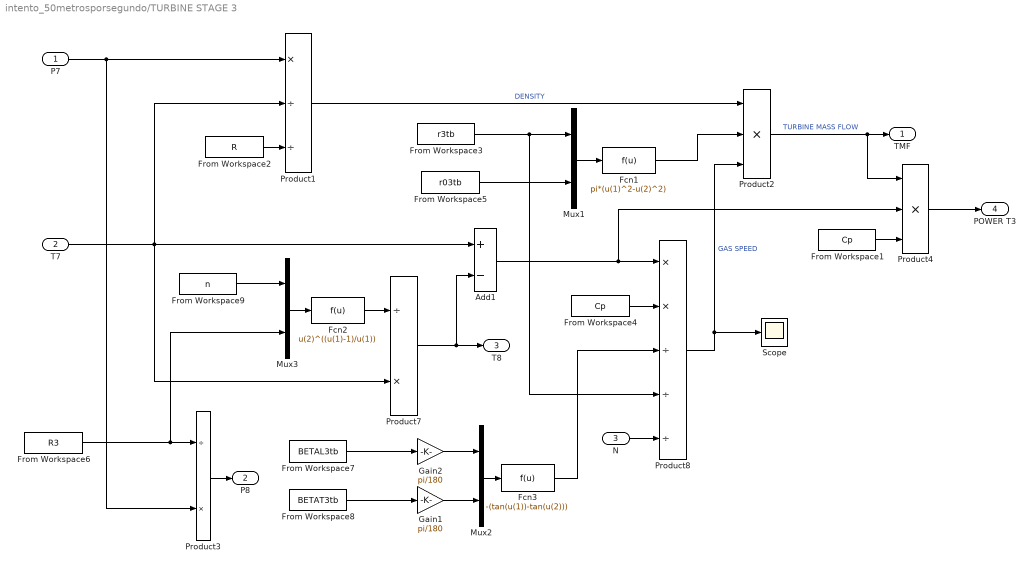
== system intento_50metrosporsegundo/TURBINE STAGE 3 ==
  P7 : Inport
  T7 : Inport  Port=2
  N : Inport  Port=3
  Add1 : Sum  Inputs=+-
  Fcn1 : Fcn  Expr=pi*(u(1)^2-u(2)^2)
  Fcn2 : Fcn  Expr=u(2)^((u(1)-1)/u(1))
  Fcn3 : Fcn  Expr=-(tan(u(1))-tan(u(2)))
  From Workspace1 : FromWorkspace  VariableName=Cp
  From Workspace2 : FromWorkspace  VariableName=R
  From Workspace3 : FromWorkspace  VariableName=r3tb
  From Workspace4 : FromWorkspace  VariableName=Cp
  From Workspace5 : FromWorkspace  VariableName=r03tb
  From Workspace6 : FromWorkspace  VariableName=R3
  From Workspace7 : FromWorkspace  VariableName=BETAL3tb
  From Workspace8 : FromWorkspace  VariableName=BETAT3tb
  From Workspace9 : FromWorkspace  VariableName=n
  Gain1 : Gain  Gain=pi/180
  Gain2 : Gain  Gain=pi/180
  Mux1 : Mux  Inputs=2
  Mux2 : Mux  Inputs=2
  Mux3 : Mux  Inputs=2
  Product1 : Product  Inputs=*//
  Product2 : Product  Inputs=3
  Product3 : Product  Inputs=/*
  Product4 : Product  Inputs=3
  Product7 : Product  Inputs=/*
  Product8 : Product  Inputs=**///
  Scope : Scope
  TMF : Outport
  P8 : Outport  Port=2
  T8 : Outport  Port=3
  POWER T3 : Outport  Port=4
  wires:
  From Workspace3/1 -> Mux1/1, Product8/4
  Mux1/1 -> Fcn1/1
  Fcn1/1 -> Product2/2
  From Workspace5/1 -> Mux1/2
  Mux2/1 -> Fcn3/1
  Gain1/1 -> Mux2/2
  From Workspace8/1 -> Gain1/1
  From Workspace7/1 -> Gain2/1
  Gain2/1 -> Mux2/1
  From Workspace2/1 -> Product1/3
  P7/1 -> Product3/2, Product1/1
  Fcn3/1 -> Product8/3
  Product3/1 -> P8/1
  From Workspace6/1 -> Product3/1, Mux3/2
  T7/1 -> Product1/2, Product7/2, Add1/1
  From Workspace9/1 -> Mux3/1
  Product7/1 -> Add1/2, T8/1
  Add1/1 -> Product4/2, Product8/1
  From Workspace4/1 -> Product8/2
  N/1 -> Product8/5
  Product8/1 -> Scope/1, Product2/3  "GAS SPEED"
  Product1/1 -> Product2/1  "DENSITY"
  Product2/1 -> Product4/1, TMF/1  "TURBINE MASS FLOW"
  Mux3/1 -> Fcn2/1
  Fcn2/1 -> Product7/1
  From Workspace1/1 -> Product4/3
  Product4/1 -> POWER T3/1

== matlab function intento_50metrosporsegundo/TRAUBS ==
  data: DENSIDAD input; Q output; velocidad_rpm input; angulo_ajuste input; velocidad_inf input; VISC input; T output; ALFA_INF output; ALFA_ATAQUE output
function [Q,T,ALFA_INF,ALFA_ATAQUE]      = fcn(DENSIDAD,velocidad_rpm,angulo_ajuste,velocidad_inf,VISC)

 ...........................PARAMETROS INICIALES ...........................
numero_de_palas=4;                  %NUMERO DE PALAS QUE TIENE EL PROPELLER
radio_maxima_pala= 0.9;              %RADIO MAXIMO DE LA PALA DEL PROPELLER
radio_base_pala=0.2;                %RADIO EN LA BASE DE LA PALA DEL PROPELLER
                           %AXIAL INFLOW FACTOR  (INITIAL)
densidad_aire=DENSIDAD;                %DENSIDAD AIRE EN KG/M^3
viscosidad_aire = VISC;            %VICOSIDAD AIRE

numero_de_divisiones=10;            %DIVISIONES QUE SE ESTIMAN PARA LA PALA %%%%%%%%%%%%%%%%%%%%%%%%%%%%%%%%%%%%%%%%%%%%%%%%%%%%%%%%%%%%Parametro que se debe cambiar
STEP_pala=(radio_maxima_pala-radio_base_pala)/numero_de_divisiones ;%STEP DEL RADIO
PALA=[radio_base_pala:STEP_pala:radio_maxima_pala]' ; % DIVISION DE LAS PALAS
tip_pala_por_divisiones = PALA(1:numero_de_divisiones,1);
theta_inicial=angulo_ajuste;                   %ANGULO GEOMETRICO DEL PROPELLER EN LA BASE
theta_final=34.5+angulo_ajuste;

STEP_theta=(theta_final-theta_inicial)/(numero_de_divisiones-1) ;%STEP DEL ANGULO 
THETA=[theta_inicial:STEP_theta:theta_final]'*pi/180;  %DIVISION DE ANGULO
THETA_FINAL=max(size(THETA));

velocidad_radianes=velocidad_rpm;

..............................TRAUBS MODEL..... ...........................
F_LOOSE=zeros(max(size(tip_pala_por_divisiones)),1);
ALFA_INF=zeros(max(size(tip_pala_por_divisiones)),1);
ALFA_ZL =[7.505656337*pi/180; 7.779161701*pi/180; 7.933172122*pi/180; 5.95941933*pi/180; 4.0123542*pi/180];%%%%%%%%%%%%%%%%%%%%%%%%%%%%%%%%%%%%%%%%%%%%%%%%%%%%%%%%%%%%Parametro que se debe cambiar
sections = [0 1 2 3 4];
degree = 4;  % Ajustar a polinomio de grado 2 (puedes cambiar el grado si lo necesitas)
p = polyfit(sections, ALFA_ZL, degree); % Ajusta un polinomio de grado 'degree'
new_sections = linspace(0, 4, max(size(tip_pala_por_divisiones))); % Genera 100 secciones intermedias
ALFA_ZL = polyval(p, new_sections); % Evalúa el polinomio ajustado en las nuevas secciones


ALFA_IND=zeros(max(size(tip_pala_por_divisiones)),1);
ALFA_ATAQUE=zeros(max(size(tip_pala_por_divisiones)),1);
CHORD=zeros(max(size(tip_pala_por_divisiones)),1);
for i=1:max(size(tip_pala_por_divisiones))
    blade_percentage=tip_pala_por_divisiones(i,1)/radio_maxima_pala;
    CHORD(i,1)=0.683*blade_percentage^5 - 3.6366*blade_percentage^4 + 6.4743*blade_percentage^3 - 5.4877*blade_percentage^2 + 2.2428*blade_percentage - 0.177;
end

CL_ALFA =[0.0846*180/pi; 0.07462*180/pi; 0.07911*180/pi; 0.08*180/pi; 0.09759*180/pi];%%%%%%%%%%%%%%%%%%%%%%%%%%%%%%%%%%%%%%%%%%%%%%%%%%%%%%%%%%%%Parametro que se debe cambiar
sections = [0 1 2 3 4];
degree = 4;  % Ajustar a polinomio de grado 2 (puedes cambiar el grado si lo necesitas)
p = polyfit(sections, CL_ALFA, degree); % Ajusta un polinomio de grado 'degree'
new_sections = linspace(0, 4, max(size(tip_pala_por_divisiones))); % Genera 100 secciones intermedias
CL_ALFA = polyval(p, new_sections); % Evalúa el polinomio ajustado en las nuevas secciones
ALFA_STALL=[14*pi/180; 12*pi/180; 6.1059*pi/180; 5.03731*pi/180; 4.6125*pi/180];
sections = [0 1 2 3 4];
degree = 4;  % Ajustar a polinomio de grado 2 (puedes cambiar el grado si lo necesitas)
p = polyfit(sections, ALFA_STALL, degree); % Ajusta un polinomio de grado 'degree'
new_sections = linspace(0, 4, max(size(tip_pala_por_divisiones))); % Genera 100 secciones intermedias
ALFA_STALL = polyval(p, new_sections); % Evalúa el polinomio ajustado en las nuevas secciones

X_ARREGLO=zeros(max(size(tip_pala_por_divisiones)),1);
sigma=1.5;
m=1.5;


CL_CORRECCION=zeros(max(size(tip_pala_por_divisiones)),1);
CD_CORRECCION=zeros(max(size(tip_pala_por_divisiones)),1);
REYNOLDS=zeros(max(size(tip_pala_por_divisiones)),1);


Kp_0 = [2.16E-37, -1.11E-30, 2.28E-24, -2.35E-18, 1.27E-12, -3.45E-07, 4.71E-02];
Kp_1 = [7.20E-38, -3.81E-31, 8.10E-25, -8.84E-19, 5.29E-13, -1.79E-07, 4.06E-02];
Kp_2 = [6.99E-38, -4.12E-31, 9.53E-25, -1.10E-18, 6.65E-13, -2.10E-07, 4.02E-02];
Kp_3 = [5.99E-38, -4.00E-31, 1.04E-24, -1.34E-18, 8.90E-13, -3.01E-07, 5.36E-02];
Kp_4 = [1.87E-38, -1.34E-31, 3.76E-25, -5.22E-19, 3.71E-13, -1.28E-07, 2.54E-02];
Kp = {Kp_0,  Kp_1, Kp_2, Kp_3, Kp_4};
Kp_new=fcn_1 (Kp);

Cdmin_0=[3.58E-37, -1.80E-30, 3.55E-24, -3.43E-18, 1.68E-12, -3.80E-07, 4.08E-02];
Cdmin_1=[2.61E-37, -1.32E-30, 2.62E-24, -2.59E-18, 1.33E-12, -3.35E-07, 4.05E-02];
Cdmin_2=[1.33E-37, -7.51E-31, 1.67E-24, -1.85E-18, 1.06E-12, -2.99E-07, 3.96E-02];
Cdmin_3=[2.23E-38, -1.52E-31, 4.11E-25, -5.60E-19, 4.08E-13, -1.56E-07, 3.21E-02];
Cdmin_4=[2.62E-38, -1.85E-31, 5.06E-25, -6.78E-19, 4.59E-13, -1.47E-07, 2.54E-02];
Cdmin = {Cdmin_0,  Cdmin_1, Cdmin_2, Cdmin_3, Cdmin_4};
Cdmin_new=fcn_1 (Cdmin);

Clmd_0=[7.64E-36, -3.55E-29, 6.37E-23, -5.64E-17, 2.61E-11, -6.01E-06, 1.03E+00];
Clmd_1=[-1.02E-36, 5.04E-30, -8.94E-24, 6.63E-18, -1.54E-12, -5.05E-07, 8.86E-01];
Clmd_2=[-2.76E-36, 1.29E-29, -2.24E-23, 1.80E-17, -6.48E-12, 5.43E-07, 7.77E-01];
Clmd_3=[-5.53E-37, 3.39E-30, -7.86E-24, 8.61E-18, -4.53E-12, 9.75E-07, 7.18E-01];
Clmd_4=[1.49E-37, -5.22E-31, -2.95E-25, 3.16E-18, -4.49E-12, 2.46E-06, -6.54E-02];
Clmd = {Clmd_0,  Clmd_1, Clmd_2, Clmd_3, Clmd_4};
Clmd_new=fcn_1 (Clmd);

function [s]= fcn_1 (Structure)
    for i=1:1:7
        arreglo=zeros(1,5);
        for j=1:1:5
            arreglo(1,j)=Structure{j}(i);
        end
        sections = [0 1 2 3 4];
        degree = 4;  % Ajustar a polinomio de grado 2 (puedes cambiar el grado si lo necesitas)
        p = polyfit(sections, arreglo, degree); % Ajusta un polinomio de grado 'degree'
        new_sections = linspace(0, 4, max(size(tip_pala_por_divisiones))); % Genera 100 secciones intermedias
        predicted_a6 = polyval(p, new_sections); % Evalúa el polinomio ajustado en las nuevas secciones
        s = zeros(max(size(tip_pala_por_divisiones)),7);
        for k=1:1:max(size(tip_pala_por_divisiones))
            s(k,i)=predicted_a6(k);
        end
    end
end


integrand1 = zeros(1,max(size(tip_pala_por_divisiones)));
integrand2 = zeros(1,max(size(tip_pala_por_divisiones)));

alfa_geometrico=  linspace(0,0,max(size(tip_pala_por_divisiones)));%linspace(0,34.5,max(size(tip_pala_por_divisiones)));
for i=1:max(size(tip_pala_por_divisiones))
        THETA(THETA_FINAL,1);
        F_LOOSE(i,1)=(2/pi)*acos(exp((-numero_de_palas*(1-tip_pala_por_divisiones(i,1)/radio_maxima_pala))/2*sin(THETA(THETA_FINAL,1))));
        ALFA_INF(i,1)=atan(velocidad_inf/(tip_pala_por_divisiones(i,1)*velocidad_radianes));
        A_CUADRATICA=F_LOOSE(i,1)*(pi/2)*cos(ALFA_INF(i,1));
        primer_termino=numero_de_palas*CHORD(i,1)*CL_ALFA(i)/(16*tip_pala_por_divisiones(i,1));
        segundo_termino=F_LOOSE(i,1)*pi*sin(ALFA_INF(i,1))/2;
        B_CUADRATICA=primer_termino+segundo_termino;
        C_CUADRATICA=-numero_de_palas*CHORD(i,1)*CL_ALFA(i)*(THETA(i,1)-ALFA_INF(i,1)-ALFA_ZL(i))/(16*tip_pala_por_divisiones(i,1));
        ALFA_IND(i,1)=(-B_CUADRATICA+sqrt(B_CUADRATICA^2-4*A_CUADRATICA*C_CUADRATICA))/(2*A_CUADRATICA);
        ALFA_ATAQUE(i,1)= THETA(i,1)-ALFA_IND(i,1)-ALFA_INF(i,1);
        X_ARREGLO(i,1)=1/(1+exp(sigma*(ALFA_ATAQUE(i,1)-ALFA_STALL(i))));
        CL_CORRECCION(i,1)=CL_ALFA(i)*ALFA_ATAQUE(i,1)*((1+X_ARREGLO(i,1)^m)/2)^2;
        REYNOLDS(i,1)=velocidad_radianes*tip_pala_por_divisiones(i,1)*cos(ALFA_IND(i,1))*densidad_aire*CHORD(i,1)/(cos(ALFA_INF(i,1))*viscosidad_aire);
        
        Kp_iterado=[Kp_new(i,1),Kp_new(i,2),Kp_new(i,3),Kp_new(i,4),Kp_new(i,5),Kp_new(i,6),Kp_new(i,7)];
        %Kp_iterado=[Kp{i}(1),Kp{i}(2),Kp{i}(3),Kp{i}(4),Kp{i}(5),Kp{i}(6),Kp{i}(7)];        
        Kp_local=polyval(Kp_iterado, REYNOLDS(i,1));

        Cdmin_iterado=[Cdmin_new(i,1),Cdmin_new(i,2),Cdmin_new(i,3),Cdmin_new(i,4),Cdmin_new(i,5),Cdmin_new(i,6),Cdmin_new(i,7)];
        %Cdmin_iterado=[Cdmin{i}(1),Cdmin{i}(2),Cdmin{i}(3),Cdmin{i}(4),Cdmin{i}(5),Cdmin{i}(6),Cdmin{i}(7)];
        Cdmin_local=polyval(Cdmin_iterado, REYNOLDS(i,1));

        Clmd_iterado=[Clmd_new(i,1),Clmd_new(i,2),Clmd_new(i,3),Clmd_new(i,4),Clmd_new(i,5),Clmd_new(i,6),Clmd_new(i,7)];
        %Clmd_iterado=[Clmd{i}(1),Clmd{i}(2),Clmd{i}(3),Clmd{i}(4),Clmd{i}(5),Clmd{i}(6),Clmd{i}(7)];
        Clmd_local=polyval(Clmd_iterado, REYNOLDS(i,1));
        
        
        CD_CORRECCION(i,1)=X_ARREGLO(i,1)*(Cdmin_local+Kp_local*(CL_CORRECCION(i,1)-Clmd_local)^2)+(1-X_ARREGLO(i,1))*(CL_CORRECCION(i,1)*tan(ALFA_ATAQUE(i,1))+0.5*Cdmin_local*cos(alfa_geometrico(i)*pi/180));
        integrand1(i)=(tip_pala_por_divisiones(i)^3 * CHORD(i,1) * cos(ALFA_IND(i,1))^2 / (cos(ALFA_INF(i,1))^2 * CL_CORRECCION(i,1))) *(sin(ALFA_IND(i,1) + ALFA_INF(i,1)) + (CD_CORRECCION(i,1) / CL_CORRECCION(i,1)) * cos(ALFA_IND(i,1) + ALFA_INF(i,1)));
        integrand2(i)=(tip_pala_por_divisiones(i)^2 * CHORD(i,1) * cos(ALFA_IND(i,1))^2 / (cos(ALFA_INF(i,1))^2 * CL_CORRECCION(i,1))) *(cos(ALFA_IND(i,1) + ALFA_INF(i,1)) - (CD_CORRECCION(i,1) / CL_CORRECCION(i,1)) * sin(ALFA_IND(i,1) + ALFA_INF(i,1)));
end
degree = 2;  % Ajustar a polinomio de grado 2 (puedes cambiar el grado si lo necesitas)
p = polyfit(tip_pala_por_divisiones, integrand1, degree); % Ajusta un polinomio de grado 'degree'
q = polyfit(tip_pala_por_divisiones, integrand2, degree);
%integrand1_1 = polyval(p, tip_pala_por_divisiones); % Evalúa el polinomio ajustado en las nuevas secciones

%integrand1_1 = @(r) p(1)*r.^5 +p(2)*r.^4 +p(3)*r.^3 +p(4)*r.^2 + p(5)*r + p(6);
%integrand1_1 = @(r) p(1)*r.^7 +p(2)*r.^6 +p(3)*r.^5 +p(4)*r.^4 +p(5)*r.^3 + p(6)*r.^2 + p(7)*r + p(8);
%integrand1_1 = @(r) p(1)*r.^3 +p(2)*r.^2 + p(3)*r + p(4);
%integrand1_1 = @(r) p(1)*r.^2 + p(2)*r + p(3);
integrand1_1 = @(r) p(1)*r + p(2);
%integrand1_1 = @(r) p(1)*r.^4 +p(2)*r.^3 +p(3)*r.^2 + p(4)*r + p(4);

%integrand2_1 = polyval(q, tip_pala_por_divisiones);
%integrand2_1 = @(r) q(1)*r.^5 +q(2)*r.^4 +q(3)*r.^3 +q(4)*r.^2 + q(5)*r + q(6);
%integrand2_1 = @(r) q(1)*r.^7 +q(2)*r.^6 +q(3)*r.^5 +q(4)*r.^4 +q(5)*r.^3 + q(6)*r.^2 + q(7)*r + q(8);
%integrand2_1 = @(r) q(1)*r.^3 +q(2)*r.^2 + q(3)*r + q(4);
%integrand2_1 = @(r) q(1)*r.^2 + q(2)*r + q(3);
integrand2_1 = @(r) q(1)*r + q(2);
%integrand2_1 = @(r) q(1)*r.^4 +q(2)*r.^3 +q(3)*r.^2 + q(4)*r + q(4);

Q = (numero_de_palas * densidad_aire * velocidad_radianes^2 / 2) *integral(integrand1_1, tip_pala_por_divisiones(1), tip_pala_por_divisiones(max(size(tip_pala_por_divisiones))));
T = (numero_de_palas * densidad_aire * velocidad_radianes^2 / 2) *integral(integrand2_1, tip_pala_por_divisiones(1), tip_pala_por_divisiones(max(size(tip_pala_por_divisiones))));

% % Aplicar el método de Simpson
% Q = (numero_de_palas .* densidad_aire .* velocidad_radianes.^2 ./ 2) * simpson_rule(max(size(tip_pala_por_divisiones)), integrand1);
% T = (numero_de_palas .* densidad_aire .* velocidad_radianes.^2 ./ 2) * simpson_rule(max(size(tip_pala_por_divisiones)), integrand2);
% % disp(['El valor de Q es: ', num2str(Q)]);
% % disp(['El valor de T es: ', num2str(T)]);
% 
% % Función para el método de Simpson
% function I = simpson_rule(x, y)
%     h = (x(end) - x(1)) / (length(x) - 1); % Paso
%     I = y(1) + y(end); % Sumar los extremos
% 
%     % Sumar las partes impares
%     for i = 2:2:length(y)-1
%         I = I + 4 * y(i);
%     end
% 
%     % Sumar las partes pares
%     for i = 3:2:length(y)-2
%         I = I + 2 * y(i);
%     end
% 
%     I = (I * h) / 3; % Multiplicar por h/3
% end
% 
end

== matlab function intento_50metrosporsegundo/MATLAB Function ==
  data: t input; torque_nom output
function torque_nom = torque_function(t)
    % Define el torque nominal basado en el tiempo
    if t <= 60 
        torque_nom = 2000; % Torque en carreteo (ejemplo bajo)
    elseif t > 60 && t <= 170
        torque_nom = 3000; % Torque durante el despegue (32° pitch)
    elseif t > 170 && t <= 420
        torque_nom = 2000; % Torque durante el crucero (44.5° o 48.5° pitch)
    elseif t > 420 && t <= 570
        torque_nom = 2000; % Torque durante la aproximación a aterrizaje
    elseif t > 570 && t <= 580
        torque_nom = 1000; % Torque durante la aproximación a aterrizaje
    else
        torque_nom = 500; % Torque en desaceleración después del aterrizaje
    end
end
